simulink model "FD_1doF"  (R2019b)
settings: Solver=VariableStepAuto  StartTime=0.0  StopTime=600  RelTol=1e-3
undefined symbols (not defined in the file): Dm, Dt, g, Jp, k_pitch, Mb
settings Model: Creator=laptop  LastModifiedBy=lbend
settings OptimizationCC: BlockReduction=off  DefaultParameterBehavior=Inlined  BufferReuse=off

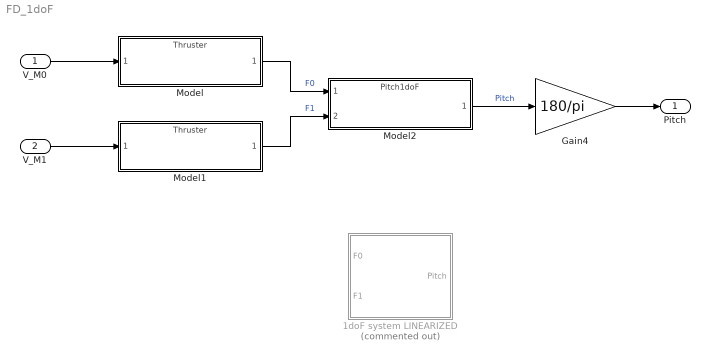
== system FD_1doF ==
  "V_M0 " : Inport
  V_M1 : Inport  Port=2
  1doF system LINEARIZED : Subsystem  Commented=on
  Gain4 : Gain  Gain=180/pi
  Model : ModelReference  ModelNameDialog=Thruster.slx  SimulationMode=Normal  ModelReferenceVersion=1.0
  Model1 : ModelReference  ModelNameDialog=Thruster.slx  SimulationMode=Normal  ModelReferenceVersion=1.0
  Model2 : ModelReference  ModelNameDialog=Pitch1doF.slx  SimulationMode=Normal  ModelReferenceVersion=1.1
  Pitch : Outport
  wires:
  Model/1 -> Model2/1  "F0"
  Model1/1 -> Model2/2  "F1"
  Model2/1 -> Gain4/1  "Pitch"
  Gain4/1 -> Pitch/1
  "V_M0 "/1 -> Model/1
  V_M1/1 -> Model1/1

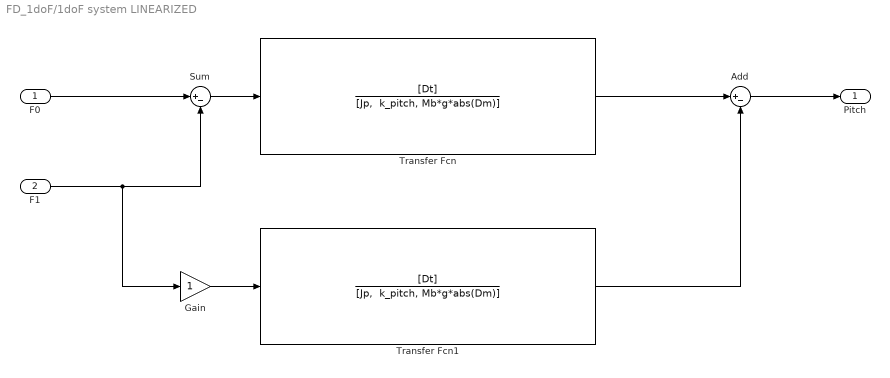
== system FD_1doF/1doF system LINEARIZED ==
  F0 : Inport
  F1 : Inport  Port=2
  Add : Sum  Inputs=|+-
  Gain : Gain
  Sum : Sum  Inputs=|+-
  Transfer Fcn : TransferFcn  Numerator=[Dt]  Denominator="[Jp,  k_pitch, Mb*g*abs(Dm)]"
  Transfer Fcn1 : TransferFcn  Numerator=[Dt]  Denominator="[Jp,  k_pitch, Mb*g*abs(Dm)]"
  Pitch : Outport
  wires:
  F0/1 -> Sum/1
  F1/1 -> Gain/1, Sum/2
  Sum/1 -> Transfer Fcn/1
  Transfer Fcn/1 -> Add/1
  Add/1 -> Pitch/1
  Transfer Fcn1/1 -> Add/2
  Gain/1 -> Transfer Fcn1/1
